simulink model "counter_to_leds"  (R2014a)
settings: Solver=FixedStepDiscrete  StartTime=0.0  StopTime=10000  FixedStep=1  RelTol=1e-3
libraries: hdlsllib x10, simulink x1
settings Model: Creator=Andrew  LastModifiedBy=ricci.an
settings OptimizationCC: BlockReduction=off  ConditionallyExecuteInputs=off  InlineParams=on
settings DebuggingCC: AlgebraicLoopMsg=error
settings HardwareCC: ProdHWDeviceType=ASIC/FPGA->ASIC/FPGA  ProdEqTarget=off

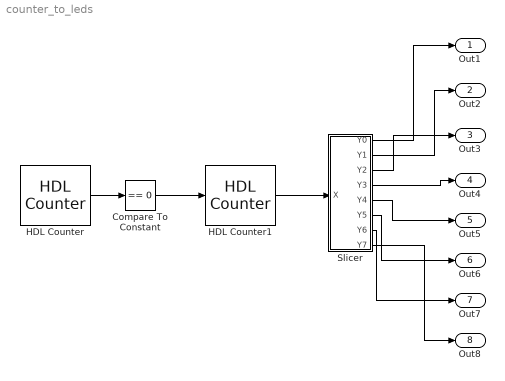
== system counter_to_leds ==
  Compare To Constant : simulink/Logic and Bit Operations/Compare To Constant  relop===  const=0  OutDataTypeStr=boolean
  HDL Counter : hdlsllib/HDL Operations/HDL Counter  CountType=Count limited  CountInit=0  CountStep=1  CountMax=25000000  CountFromType=Initial value  CountFrom=0  CountResetPort=off  CountLoadPort=off  CountEnbPort=off  CountDirPort=off  CountDataType=Unsigned  CountWordLen=32  CountFracLen=0  CountSampTime=1
  HDL Counter1 : hdlsllib/HDL Operations/HDL Counter  CountType=Free running  CountInit=0  CountStep=1  CountMax=100  CountFromType=Initial value  CountFrom=0  CountResetPort=off  CountLoadPort=off  CountEnbPort=on  CountDirPort=off  CountDataType=Unsigned  CountWordLen=8  CountFracLen=0  CountSampTime=1
  Slicer : Subsystem
  Out1 : Outport
  Out2 : Outport  Port=2
  Out3 : Outport  Port=3
  Out4 : Outport  Port=4
  Out5 : Outport  Port=5
  Out6 : Outport  Port=6
  Out7 : Outport  Port=7
  Out8 : Outport  Port=8
  wires:
  HDL Counter/1 -> Compare To Constant/1
  Compare To Constant/1 -> HDL Counter1/1
  HDL Counter1/1 -> Slicer/1(X)
  Slicer/1(Y0) -> Out1/1
  Slicer/2(Y1) -> Out2/1
  Slicer/3(Y2) -> Out3/1
  Slicer/4(Y3) -> Out4/1
  Slicer/5(Y4) -> Out5/1
  Slicer/6(Y5) -> Out6/1
  Slicer/7(Y6) -> Out7/1
  Slicer/8(Y7) -> Out8/1

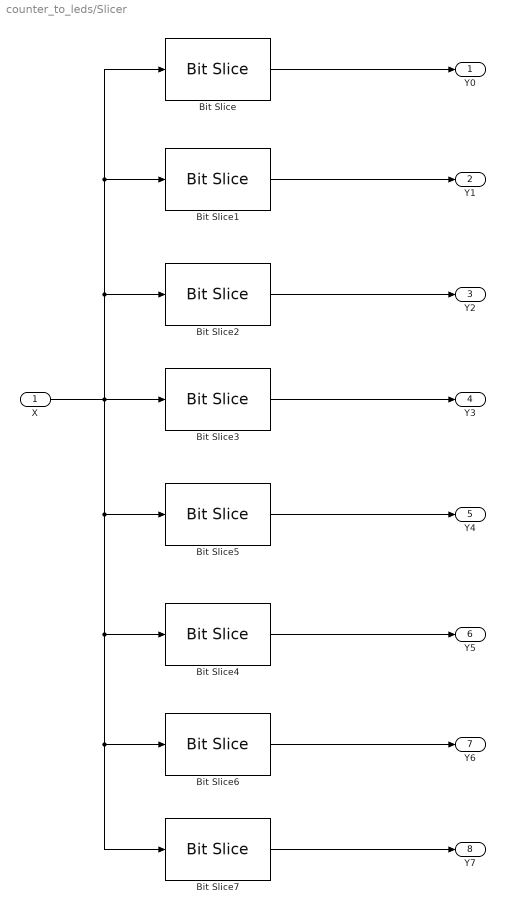
== system counter_to_leds/Slicer ==
  X : Inport  OutDataTypeStr=uint8  SampleTime=1
  Bit Slice : hdlsllib/HDL Operations/Bit Slice  lidx=7  ridx=7
  Bit Slice1 : hdlsllib/HDL Operations/Bit Slice  lidx=6  ridx=6
  Bit Slice2 : hdlsllib/HDL Operations/Bit Slice  lidx=5  ridx=5
  Bit Slice3 : hdlsllib/HDL Operations/Bit Slice  lidx=4  ridx=4
  Bit Slice4 : hdlsllib/HDL Operations/Bit Slice  lidx=2  ridx=2
  Bit Slice5 : hdlsllib/HDL Operations/Bit Slice  lidx=3  ridx=3
  Bit Slice6 : hdlsllib/HDL Operations/Bit Slice  lidx=1  ridx=1
  Bit Slice7 : hdlsllib/HDL Operations/Bit Slice  lidx=0  ridx=0
  Y0 : Outport
  Y1 : Outport  Port=2
  Y2 : Outport  Port=3
  Y3 : Outport  Port=4
  Y4 : Outport  Port=5
  Y5 : Outport  Port=6
  Y6 : Outport  Port=7
  Y7 : Outport  Port=8
  wires:
  X/1 -> Bit Slice7/1, Bit Slice6/1, Bit Slice4/1, Bit Slice5/1, Bit Slice/1, Bit Slice1/1, Bit Slice2/1, Bit Slice3/1
  Bit Slice/1 -> Y0/1
  Bit Slice7/1 -> Y7/1
  Bit Slice3/1 -> Y3/1
  Bit Slice1/1 -> Y1/1
  Bit Slice5/1 -> Y4/1
  Bit Slice2/1 -> Y2/1
  Bit Slice4/1 -> Y5/1
  Bit Slice6/1 -> Y6/1
